simulink model "Integ_Model_Hepta"  (R2022a)
settings: configuration reference "VLS_Standard_Configuration" (kept outside this file)
undefined symbols (not defined in the file or in its folder): C_AFS_SpeedThrAct, C_AfsRampTimeMatrix, C_AnimationOnLoop, C_AnimationPeriod, C_AnimationPriority, C_CieCurveGammaToPwmY, C_CieCurvePwmToGammaY, C_CL_Ti_Speed_Hystresis, C_CL_Ti_Speed_Threshold, C_ClActAlgo, C_ClLeftSideTable_Alpha1, C_ClLeftSideTable_Alpha2, C_ClManeuverPwm, C_ClRightSideTable_Alpha1, C_ClRightSideTable_Alpha2, C_ClSpeedCurve, C_ClTableSize, C_ClTownPwm, C_Config, C_CSpeed0, C_DblDeadZone, C_DblEnable, C_DblInterDblAngValues, C_DblInterStwAngValues, C_DblLeftAngles, C_DblRampTime, C_DblRateLimit, C_DblRightAngles, C_DblSlavePeriod, C_DblSpeed0, C_DefaultValue, C_DrlRampTime, C_EndIndexOfEachLightingModule, C_EndValues, C_ForceExternalAfsMode, C_IndexOfStartStepForEachScenario, C_IsClOnTps, C_IsDblActive, C_IsDrlAutorizedInPower2, C_IsDrlPlOnTps, C_IsPlAutorizedInPower2, C_IsTiAutorizedInPower2, C_IsTiOnTps, C_LedCenterDist, C_LedCenterLimits, C_LedLeftDist, C_LedRightDist, C_LedStartIndexOfCl, C_LedStartIndexOfDrlPl, C_LedStartIndexOfTi, C_LeftDblMaxAngle, C_LeftDblMinAngle, C_MaintainAnimationPwm, C_MaintainAnimationTime, C_NumOfStepsForEachScenario, C_PlNominalPwm, C_PlOverDRL, C_RightDblMaxAngle, C_RightDblMinAngle, C_StartIndexOfEachLightingModule ... (+14)
libraries: simulink x11, AFS_MasterFeature x2, DodecaPreprocessingLib x1, Cl_Lib x1, DBL_MasterLib x1, AfsSlaveLib x1, DblSlaveLib x1, StdAnimationLibrary_R2020b x1, Ramp_Library_R2017b x1, STD_Signaling_Lib x1
(part 1 of 2)
settings Model: DataDictionary=Hepta_Integrated_SLDD.sldd  Creator=ahashem  LastModifiedBy=yli69
settings ConfigSetRef: SourceName=VLS_Standard_Configuration

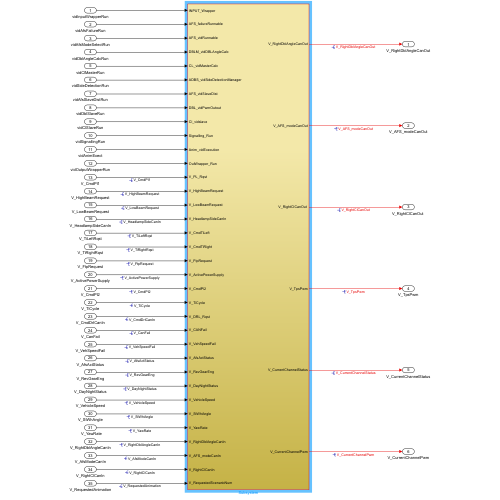
[thumbnail: Simulink's stored preview of the top-level diagram]
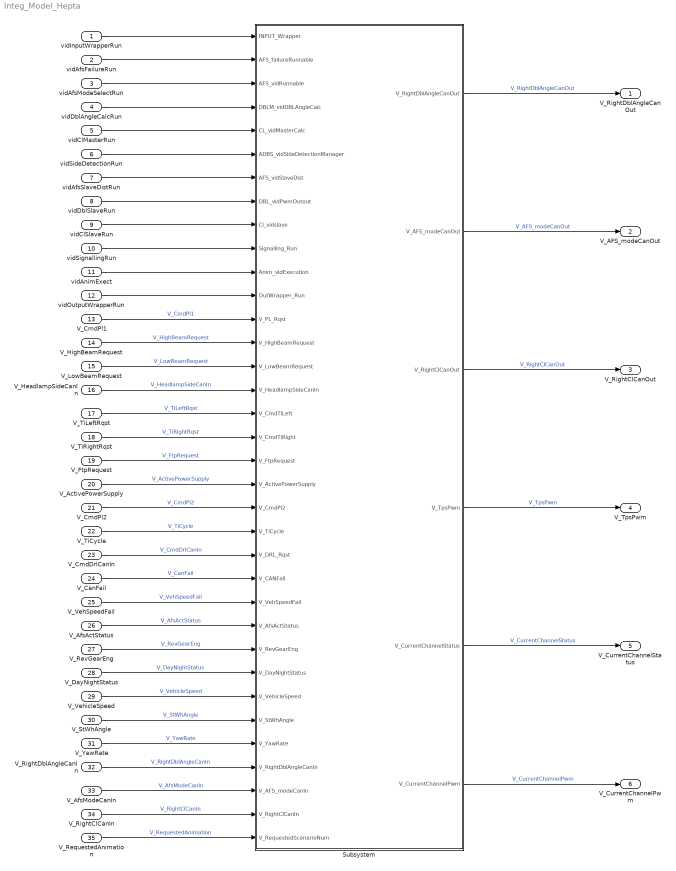
== system Integ_Model_Hepta ==
  vidInputWrapperRun : Inport  OutputFunctionCall=on
  vidAfsFailureRun : Inport  Port=2  OutputFunctionCall=on
  vidAfsModeSelectRun : Inport  Port=3  OutputFunctionCall=on
  vidDblAngleCalcRun : Inport  Port=4  SampleTime=0.02  OutputFunctionCall=on
  vidClMasterRun : Inport  Port=5  SampleTime=0.02  OutputFunctionCall=on
  vidSideDetectionRun : Inport  Port=6  OutputFunctionCall=on
  vidAfsSlaveDistRun : Inport  Port=7  OutputFunctionCall=on
  vidDblSlaveRun : Inport  Port=8  OutputFunctionCall=on
  vidClSlaveRun : Inport  Port=9  OutputFunctionCall=on
  vidSignallingRun : Inport  Port=10  OutputFunctionCall=on
  vidAnimExect : Inport  Port=11  OutputFunctionCall=on
  vidOutputWrapperRun : Inport  Port=12  OutputFunctionCall=on
  V_CmdPl1 : Inport  Port=13
  V_HighBeamRequest : Inport  Port=14
  V_LowBeamRequest : Inport  Port=15
  V_HeadlampSideCanIn : Inport  Port=16
  V_TiLeftRqst : Inport  Port=17
  V_TiRightRqst : Inport  Port=18
  V_FtpRequest : Inport  Port=19
  V_ActivePowerSupply : Inport  Port=20
  V_CmdPl2 : Inport  Port=21
  V_TiCycle : Inport  Port=22
  V_CmdDrlCanIn : Inport  Port=23
  V_CanFail : Inport  Port=24
  V_VehSpeedFail : Inport  Port=25
  V_AfsActStatus : Inport  Port=26
  V_RevGearEng : Inport  Port=27
  V_DayNightStatus : Inport  Port=28
  V_VehicleSpeed : Inport  Port=29
  V_StWhAngle : Inport  Port=30
  "  V_YawRate" : Inport  Port=31
  V_RightDblAngleCanIn : Inport  Port=32
  V_AfsModeCanIn : Inport  Port=33
  V_RightClCanIn : Inport  Port=34
  V_RequestedAnimation : Inport  Port=35
  Subsystem : Subsystem
  V_RightDblAngleCanOut : Outport  VectorParamsAs1DForOutWhenUnconnected=off
  V_AFS_modeCanOut : Outport  Port=2  VectorParamsAs1DForOutWhenUnconnected=off
  "V_RightClCanOut " : Outport  Port=3  VectorParamsAs1DForOutWhenUnconnected=off
  V_TpsPwm : Outport  Port=4
  V_CurrentChannelStatus : Outport  Port=5
  V_CurrentChannelPwm : Outport  Port=6
  wires:
  vidSignallingRun/1 -> Subsystem/10(Signalling_Run)
  vidInputWrapperRun/1 -> Subsystem/1(INPUT_Wrapper)
  vidAfsSlaveDistRun/1 -> Subsystem/7(AFS_vidSlaveDist)
  V_CmdPl1/1 -> Subsystem/13(V_PL_Rqst)  "V_CmdPl1"
  V_CmdDrlCanIn/1 -> Subsystem/23(V_DRL_Rqst)  "V_CmdDrlCanIn"
  V_HighBeamRequest/1 -> Subsystem/14(V_HighBeamRequest)  "V_HighBeamRequest"
  V_LowBeamRequest/1 -> Subsystem/15(V_LowBeamRequest)  "V_LowBeamRequest"
  vidDblSlaveRun/1 -> Subsystem/8(DBL_vidPwmOutout)
  V_HeadlampSideCanIn/1 -> Subsystem/16(V_HeadlampSideCanIn)  "V_HeadlampSideCanIn"
  V_TiRightRqst/1 -> Subsystem/18(V_CmdTiRight)  "V_TiRightRqst"
  V_TiLeftRqst/1 -> Subsystem/17(V_CmdTiLeft)  "V_TiLeftRqst"
  V_FtpRequest/1 -> Subsystem/19(V_FtpRequest)  "V_FtpRequest"
  V_ActivePowerSupply/1 -> Subsystem/20(V_ActivePowerSupply)  "V_ActivePowerSupply"
  V_TiCycle/1 -> Subsystem/22(V_TiCycle)  "V_TiCycle"
  V_CmdPl2/1 -> Subsystem/21(V_CmdPl2)  "V_CmdPl2"
  vidOutputWrapperRun/1 -> Subsystem/12(OutWrapper_Run)
  vidSideDetectionRun/1 -> Subsystem/6(ADBS_vidSideDetectionManager)
  vidAfsFailureRun/1 -> Subsystem/2(AFS_failureRunnable)
  vidAfsModeSelectRun/1 -> Subsystem/3(AFS_vidRunnable)
  vidDblAngleCalcRun/1 -> Subsystem/4(DBLM_vidDBLAngleCalc)
  V_CanFail/1 -> Subsystem/24(V_CANFail)  "V_CanFail"
  V_VehSpeedFail/1 -> Subsystem/25(V_VehSpeedFail)  "V_VehSpeedFail"
  V_AfsActStatus/1 -> Subsystem/26(V_AfsActStatus)  "V_AfsActStatus"
  V_RevGearEng/1 -> Subsystem/27(V_RevGearEng)  "V_RevGearEng"
  V_DayNightStatus/1 -> Subsystem/28(V_DayNightStatus)  "V_DayNightStatus"
  V_AfsModeCanIn/1 -> Subsystem/33(V_AFS_modeCanIn)  "V_AfsModeCanIn"
  V_RightDblAngleCanIn/1 -> Subsystem/32(V_RightDblAngleCanIn)  "V_RightDblAngleCanIn"
  V_VehicleSpeed/1 -> Subsystem/29(V_VehicleSpeed)  "V_VehicleSpeed"
  V_StWhAngle/1 -> Subsystem/30(V_StWhAngle)  "V_StWhAngle"
  "  V_YawRate"/1 -> Subsystem/31(V_YawRate)  "V_YawRate"
  Subsystem/2(V_AFS_modeCanOut) -> V_AFS_modeCanOut/1  "V_AFS_modeCanOut"
  Subsystem/1(V_RightDblAngleCanOut) -> V_RightDblAngleCanOut/1  "V_RightDblAngleCanOut"
  vidClMasterRun/1 -> Subsystem/5(CL_vidMasterCalc)
  vidClSlaveRun/1 -> Subsystem/9(Cl_vidslave)
  V_RightClCanIn/1 -> Subsystem/34(V_RightClCanIn)  "V_RightClCanIn"
  Subsystem/3("V_RightClCanOut ") -> "V_RightClCanOut "/1  "V_RightClCanOut"
  Subsystem/4(V_TpsPwm) -> V_TpsPwm/1  "V_TpsPwm"
  Subsystem/5(V_CurrentChannelStatus) -> V_CurrentChannelStatus/1  "V_CurrentChannelStatus"
  Subsystem/6(V_CurrentChannelPwm) -> V_CurrentChannelPwm/1  "V_CurrentChannelPwm"
  vidAnimExect/1 -> Subsystem/11(Anim_vidExecution)
  V_RequestedAnimation/1 -> Subsystem/35(V_RequestedScenarioNum)  "V_RequestedAnimation"

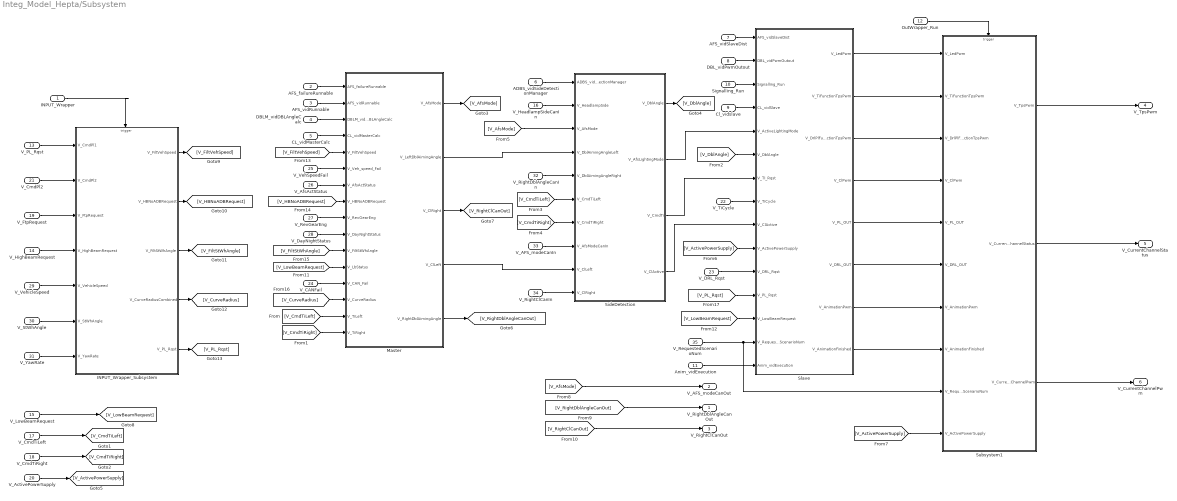
== system Integ_Model_Hepta/Subsystem ==
  INPUT_Wrapper : Inport
  AFS_failureRunnable : Inport  Port=2  OutputFunctionCall=on
  AFS_vidRunnable : Inport  Port=3  OutputFunctionCall=on
  DBLM_vidDBLAngleCalc : Inport  Port=4  SampleTime=0.02  OutputFunctionCall=on
  CL_vidMasterCalc : Inport  Port=5  SampleTime=0.02  OutputFunctionCall=on
  ADBS_vidSideDetectionManager : Inport  Port=6
  AFS_vidSlaveDist : Inport  Port=7
  DBL_vidPwmOutout : Inport  Port=8
  Cl_vidslave : Inport  Port=9
  Signalling_Run : Inport  Port=10
  Anim_vidExecution : Inport  Port=11
  OutWrapper_Run : Inport  Port=12
  V_PL_Rqst : Inport  Port=13
  V_HighBeamRequest : Inport  Port=14
  V_LowBeamRequest : Inport  Port=15
  V_HeadlampSideCanIn : Inport  Port=16
  V_CmdTiLeft : Inport  Port=17
  V_CmdTiRight : Inport  Port=18
  V_FtpRequest : Inport  Description=|  Port=19
      | Requirements:
      | Covers{PAKU_YRS_2769}
  V_ActivePowerSupply : Inport  Port=20
  V_CmdPl2 : Inport  Port=21
  V_TiCycle : Inport  Port=22
  V_DRL_Rqst : Inport  Port=23
  V_CANFail : Inport  Port=24
  V_VehSpeedFail : Inport  Port=25
  V_AfsActStatus : Inport  Port=26
  V_RevGearEng : Inport  Port=27
  V_DayNightStatus : Inport  Port=28
  V_VehicleSpeed : Inport  Port=29
  V_StWhAngle : Inport  Port=30
  V_YawRate : Inport  Port=31
  V_RightDblAngleCanIn : Inport  Port=32
  V_AFS_modeCanIn : Inport  Port=33
  V_RightClCanIn : Inport  Port=34
  V_RequestedScenarioNum : Inport  Port=35
  INPUT_Wrapper_Subsystem : Subsystem  Description=Clustering subsystem
  Master : Subsystem
  SideDetection : Subsystem
  Slave : Subsystem
  Subsystem1 : Subsystem
  V_RightDblAngleCanOut : Outport  VectorParamsAs1DForOutWhenUnconnected=off
  V_AFS_modeCanOut : Outport  Port=2  VectorParamsAs1DForOutWhenUnconnected=off
  "V_RightClCanOut " : Outport  Port=3  VectorParamsAs1DForOutWhenUnconnected=off
  V_TpsPwm : Outport  Port=4
  V_CurrentChannelStatus : Outport  Port=5
  V_CurrentChannelPwm : Outport  Port=6
  wires:
  V_LowBeamRequest/1 -> [V_LowBeamRequest]
  INPUT_Wrapper/1 -> INPUT_Wrapper_Subsystem/Trigger
  AFS_vidSlaveDist/1 -> Slave/1(AFS_vidSlaveDist)
  DBL_vidPwmOutout/1 -> Slave/2(DBL_vidPwmOutout)
  V_FtpRequest/1 -> INPUT_Wrapper_Subsystem/3(V_FtpRequest)
  V_HeadlampSideCanIn/1 -> SideDetection/2(V_HeadlampSide)
  V_CmdTiLeft/1 -> [V_CmdTiLeft]
  SideDetection/3(V_CmdTi) -> Slave/7(V_TI_Rqst)
  Slave/2(V_TiFunctionTpsPwm) -> Subsystem1/2(V_TiFunctionTpsPwm)
  Slave/3(V_DrlPlFunctionTpsPwm) -> Subsystem1/3(V_DrlPlFunctionTpsPwm)
  V_PL_Rqst/1 -> INPUT_Wrapper_Subsystem/1(V_CmdPl1)
  V_CmdPl2/1 -> INPUT_Wrapper_Subsystem/2(V_CmdPl2)
  OutWrapper_Run/1 -> Subsystem1/Trigger
  V_DRL_Rqst/1 -> Slave/11(V_DRL_Rqst)
  V_TiCycle/1 -> Slave/8(V_TiCycle)
  Signalling_Run/1 -> Slave/3(Signalling_Run)
  Slave/1(V_LedPwm) -> Subsystem1/1(V_LedPwm)
  ADBS_vidSideDetectionManager/1 -> SideDetection/1(ADBS_vidSideDetectionManager)
  Master/2(V_LeftDblAimingAngle) -> SideDetection/4(V_DblAimingAngleLeft)
  AFS_vidRunnable/1 -> Master/2(AFS_vidRunnable)
  AFS_failureRunnable/1 -> Master/1(AFS_failureRunnable)
  DBLM_vidDBLAngleCalc/1 -> Master/3(DBLM_vidDBLAngleCalc)
  V_AfsActStatus/1 -> Master/7(V_AfsActStatus)
  V_DayNightStatus/1 -> Master/10(V_DayNightStatus)
  V_CANFail/1 -> Master/13(V_CAN_Fail)
  V_VehSpeedFail/1 -> Master/6(V_Veh_speed_Fail)
  V_RevGearEng/1 -> Master/9(V_RevGearEng)
  V_HighBeamRequest/1 -> INPUT_Wrapper_Subsystem/4(V_HighBeamRequest)
  Master/1(V_AfsMode) -> [V_AfsMode]
  SideDetection/2(V_AfsLightingMode) -> Slave/5(V_ActiveLightingMode)
  V_RightDblAngleCanIn/1 -> SideDetection/5(V_DblAimingAngleRight)
  V_AFS_modeCanIn/1 -> SideDetection/8(V_AfsModeCanIn)
  V_StWhAngle/1 -> INPUT_Wrapper_Subsystem/6(V_StWhAngle)
  V_YawRate/1 -> INPUT_Wrapper_Subsystem/7(V_YawRate)
  V_VehicleSpeed/1 -> INPUT_Wrapper_Subsystem/5(V_VehicleSpeed)
  Master/4(V_ClLeft) -> SideDetection/9(V_ClLeft)
  V_RightClCanIn/1 -> SideDetection/10(V_ClRight)
  SideDetection/4(V_ClActive) -> Slave/9(V_ClActive)
  Cl_vidslave/1 -> Slave/4(CL_vidSlave)
  CL_vidMasterCalc/1 -> Master/4(CL_vidMasterCalc)
  V_CmdTiRight/1 -> [V_CmdTiRight]
  [V_CmdTiLeft] -> Master/15(V_TiLeft)
  [V_CmdTiRight] -> Master/16(V_TiRight)
  [V_AfsMode] -> SideDetection/3(V_AfsMode)
  [V_CmdTiLeft] -> SideDetection/6(V_CmdTiLeft)
  [V_CmdTiRight] -> SideDetection/7(V_CmdTiRight)
  SideDetection/1(V_DblAngle) -> [V_DblAngle]
  [V_DblAngle] -> Slave/6(V_DblAngle)
  V_ActivePowerSupply/1 -> [V_ActivePowerSupply]
  [V_ActivePowerSupply] -> Slave/10(V_ActivePowerSupply)
  [V_ActivePowerSupply] -> Subsystem1/10(V_ActivePowerSupply)
  [V_AfsMode] -> V_AFS_modeCanOut/1
  Master/5(V_RightDblAimingAngle) -> [V_RightDblAngleCanOut]
  [V_RightDblAngleCanOut] -> V_RightDblAngleCanOut/1
  Master/3(V_ClRight) -> [V_RightClCanOut]
  [V_RightClCanOut] -> "V_RightClCanOut "/1
  Subsystem1/3(V_CurrentChannelPwm) -> V_CurrentChannelPwm/1
  Subsystem1/2(V_CurrentChannelStatus) -> V_CurrentChannelStatus/1
  Subsystem1/1(V_TpsPwm) -> V_TpsPwm/1
  Slave/5(V_PL_OUT) -> Subsystem1/5(V_PL_OUT)
  Slave/6(V_DRL_OUT) -> Subsystem1/6(V_DRL_OUT)
  Slave/4(V_ClPwm) -> Subsystem1/4(V_ClPwm)
  [V_LowBeamRequest] -> Master/12(V_LbStatus)
  [V_LowBeamRequest] -> Slave/13(V_LowBeamRequest)
  Anim_vidExecution/1 -> Slave/15(Anim_vidExecution)
  Slave/7(V_AnimationPwm) -> Subsystem1/7(V_AnimationPwm)
  Slave/8(V_AnimationFinished) -> Subsystem1/8(V_AnimationFinished)
  V_RequestedScenarioNum/1 -> Subsystem1/9(V_RequestedScenarioNum), Slave/14(V_RequestedScenarioNum)
  INPUT_Wrapper_Subsystem/1(V_FiltVehSpeed) -> [V_FiltVehSpeed]
  [V_FiltVehSpeed] -> Master/5(V_FiltVehSpeed)
  INPUT_Wrapper_Subsystem/2(V_HBNoADBRequest) -> [V_HBNoADBRequest]
  [V_HBNoADBRequest] -> Master/8(V_HBNoADBRequest)
  INPUT_Wrapper_Subsystem/3(V_FiltStWhAngle) -> [V_FiltStWhAngle]
  [V_FiltStWhAngle] -> Master/11(V_FiltStWhAngle)
  INPUT_Wrapper_Subsystem/4(V_CurveRadiusCombined) -> [V_CurveRadius]
  [V_CurveRadius] -> Master/14(V_CurveRadius)
  INPUT_Wrapper_Subsystem/5(V_PL_Rqst) -> [V_PL_Rqst]
  [V_PL_Rqst] -> Slave/12(V_PL_Rqst)

== system Integ_Model_Hepta/Subsystem/INPUT_Wrapper_Subsystem ==
  V_CmdPl1 : Inport
  V_CmdPl2 : Inport  Port=2
  V_FtpRequest : Inport  Port=3
  V_HighBeamRequest : Inport  Port=4
  V_VehicleSpeed : Inport  Port=5
  V_StWhAngle : Inport  Port=6
  V_YawRate : Inport  Port=7
  function : TriggerPort  TriggerType=function-call  VariantControl=Variant
      settings: AttributesFormatString=StatesWhenEnabling: %<StatesWhenEnabling>
  DodecaPreprocessingLib : DodecaPreprocessingLib/DodecaPreprocessingLib  SystemSampleTime=-1  VariantActivationTime=update diagram  Latency=0  AutoFrameSizeCalculation=off
  Logical Operator1 : Logic  Operator=OR  AllPortsSameDT=off  OutDataTypeStr=boolean
  Logical Operator2 : Logic  Operator=OR  AllPortsSameDT=off  OutDataTypeStr=boolean
  Terminator : Terminator
  Terminator1 : Terminator
  Terminator2 : Terminator
  V_FiltVehSpeed : Outport  VectorParamsAs1DForOutWhenUnconnected=off
  V_HBNoADBRequest : Outport  Port=2
  V_FiltStWhAngle : Outport  Port=3  VectorParamsAs1DForOutWhenUnconnected=off
  V_CurveRadiusCombined : Outport  Port=4  VectorParamsAs1DForOutWhenUnconnected=off
  V_PL_Rqst : Outport  Port=5
  wires:
  V_CmdPl1/1 -> Logical Operator2/1
  V_CmdPl2/1 -> Logical Operator2/2
  Logical Operator2/1 -> V_PL_Rqst/1
  V_FtpRequest/1 -> Logical Operator1/1
  V_HighBeamRequest/1 -> Logical Operator1/2
  Logical Operator1/1 -> V_HBNoADBRequest/1
  V_VehicleSpeed/1 -> DodecaPreprocessingLib/1
  V_StWhAngle/1 -> DodecaPreprocessingLib/2
  V_YawRate/1 -> DodecaPreprocessingLib/3
  DodecaPreprocessingLib/3 -> Terminator/1
  DodecaPreprocessingLib/4 -> Terminator1/1
  DodecaPreprocessingLib/5 -> Terminator2/1
  DodecaPreprocessingLib/2 -> V_FiltStWhAngle/1
  DodecaPreprocessingLib/1 -> V_FiltVehSpeed/1
  DodecaPreprocessingLib/6 -> V_CurveRadiusCombined/1

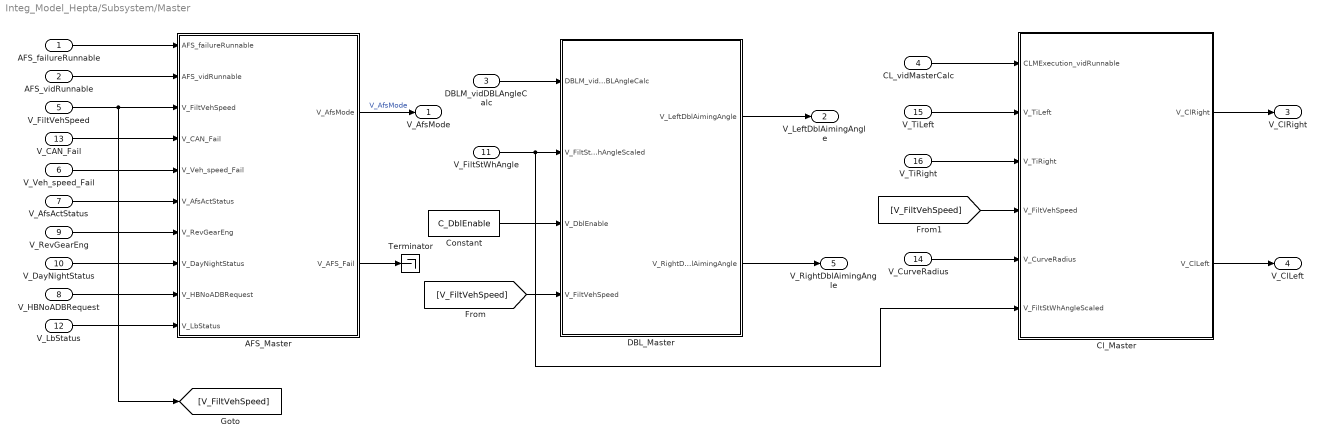
== system Integ_Model_Hepta/Subsystem/Master ==
  AFS_failureRunnable : Inport  OutputFunctionCall=on
  AFS_vidRunnable : Inport  Port=2  OutputFunctionCall=on
  DBLM_vidDBLAngleCalc : Inport  Port=3  SampleTime=0.02  OutputFunctionCall=on
  CL_vidMasterCalc : Inport  Port=4  SampleTime=0.02  OutputFunctionCall=on
  V_FiltVehSpeed : Inport  Port=5
  V_Veh_speed_Fail : Inport  Port=6
  V_AfsActStatus : Inport  Port=7
  V_HBNoADBRequest : Inport  Port=8
  V_RevGearEng : Inport  Port=9
  V_DayNightStatus : Inport  Port=10
  V_FiltStWhAngle : Inport  Port=11
  V_LbStatus : Inport  Port=12
  V_CAN_Fail : Inport  Port=13
  V_CurveRadius : Inport  Port=14
  V_TiLeft : Inport  Port=15
  V_TiRight : Inport  Port=16
  AFS_Master : Subsystem
  Cl_Master : Subsystem
  Constant : Constant  Value=C_DblEnable  OutDataTypeStr=Inherit: Inherit via back propagation
  DBL_Master : Subsystem
  Terminator : Terminator
  V_AfsMode : Outport  PortDimensions=1
  V_LeftDblAimingAngle : Outport  Port=2  VectorParamsAs1DForOutWhenUnconnected=off
  V_ClRight : Outport  Port=3
  V_ClLeft : Outport  Port=4
  V_RightDblAimingAngle : Outport  Port=5  VectorParamsAs1DForOutWhenUnconnected=off
  wires:
  AFS_Master/2(V_AFS_Fail) -> Terminator/1
  AFS_Master/1(V_AfsMode) -> V_AfsMode/1  "V_AfsMode"
  AFS_failureRunnable/1 -> AFS_Master/1(AFS_failureRunnable)
  AFS_vidRunnable/1 -> AFS_Master/2(AFS_vidRunnable)
  V_FiltVehSpeed/1 -> [V_FiltVehSpeed], AFS_Master/3(V_FiltVehSpeed)
  V_CAN_Fail/1 -> AFS_Master/4(V_CAN_Fail)
  V_Veh_speed_Fail/1 -> AFS_Master/5(V_Veh_speed_Fail)
  V_AfsActStatus/1 -> AFS_Master/6(V_AfsActStatus)
  V_FiltStWhAngle/1 -> Cl_Master/6(V_FiltStWhAngleScaled), DBL_Master/2(V_FiltStWhAngleScaled)
  Constant/1 -> DBL_Master/3(V_DblEnable)
  DBLM_vidDBLAngleCalc/1 -> DBL_Master/1(DBLM_vidDBLAngleCalc)
  DBL_Master/1(V_LeftDblAimingAngle) -> V_LeftDblAimingAngle/1
  DBL_Master/2(V_RightDblAimingAngle) -> V_RightDblAimingAngle/1
  Cl_Master/2(V_ClLeft) -> V_ClLeft/1
  V_TiLeft/1 -> Cl_Master/2(V_TiLeft)
  CL_vidMasterCalc/1 -> Cl_Master/1(CLMExecution_vidRunnable)
  V_TiRight/1 -> Cl_Master/3(V_TiRight)
  V_CurveRadius/1 -> Cl_Master/5(V_CurveRadius)
  Cl_Master/1(V_ClRight) -> V_ClRight/1
  V_RevGearEng/1 -> AFS_Master/7(V_RevGearEng)
  V_DayNightStatus/1 -> AFS_Master/8(V_DayNightStatus)
  V_HBNoADBRequest/1 -> AFS_Master/9(V_HBNoADBRequest)
  V_LbStatus/1 -> AFS_Master/10(V_LbStatus)
  [V_FiltVehSpeed] -> DBL_Master/4(V_FiltVehSpeed)
  [V_FiltVehSpeed] -> Cl_Master/4(V_FiltVehSpeed)

== system Integ_Model_Hepta/Subsystem/SideDetection ==
  ADBS_vidSideDetectionManager : Inport
  V_HeadlampSide : Inport  Port=2
  V_AfsMode : Inport  Port=3
  V_DblAimingAngleLeft : Inport  Port=4
  V_DblAimingAngleRight : Inport  Port=5
  V_CmdTiLeft : Inport  Port=6
  V_CmdTiRight : Inport  Port=7
  V_AfsModeCanIn : Inport  Port=8
  V_ClLeft : Inport  Port=9
  V_ClRight : Inport  Port=10
  SideDetectionManager : Subsystem  Description=|
      | Requirements:
      | Covers{PAKU_YRS_2708,PAKU_YRS_2758,PAKU_YRS_2734,PAKU_YRS_2753,PAKU_YRS_2783}
  V_DblAngle : Outport
  V_AfsLightingMode : Outport  Port=2
  V_CmdTi : Outport  Port=3
  V_ClActive : Outport  Port=4
  wires:
  ADBS_vidSideDetectionManager/1 -> SideDetectionManager/Trigger
  V_HeadlampSide/1 -> SideDetectionManager/1(V_HeadlampSide)
  V_DblAimingAngleLeft/1 -> SideDetectionManager/2(V_DblAimingAngleLeft)
  V_CmdTiLeft/1 -> SideDetectionManager/4(V_CmdTiLeft)
  V_DblAimingAngleRight/1 -> SideDetectionManager/3(V_DblAimingAngleRight)
  V_CmdTiRight/1 -> SideDetectionManager/5(V_CmdTiRight)
  SideDetectionManager/2(V_DblAngle) -> V_DblAngle/1
  SideDetectionManager/3(V_CmdTi) -> V_CmdTi/1
  V_AfsMode/1 -> SideDetectionManager/6(V_AfsMode)
  V_AfsModeCanIn/1 -> SideDetectionManager/7(V_AfsModeCanIn)
  SideDetectionManager/1(V_AfsLightingMode) -> V_AfsLightingMode/1
  V_ClLeft/1 -> SideDetectionManager/8(V_ClLeft)
  V_ClRight/1 -> SideDetectionManager/9(V_ClRight)
  SideDetectionManager/4(V_ClActive) -> V_ClActive/1

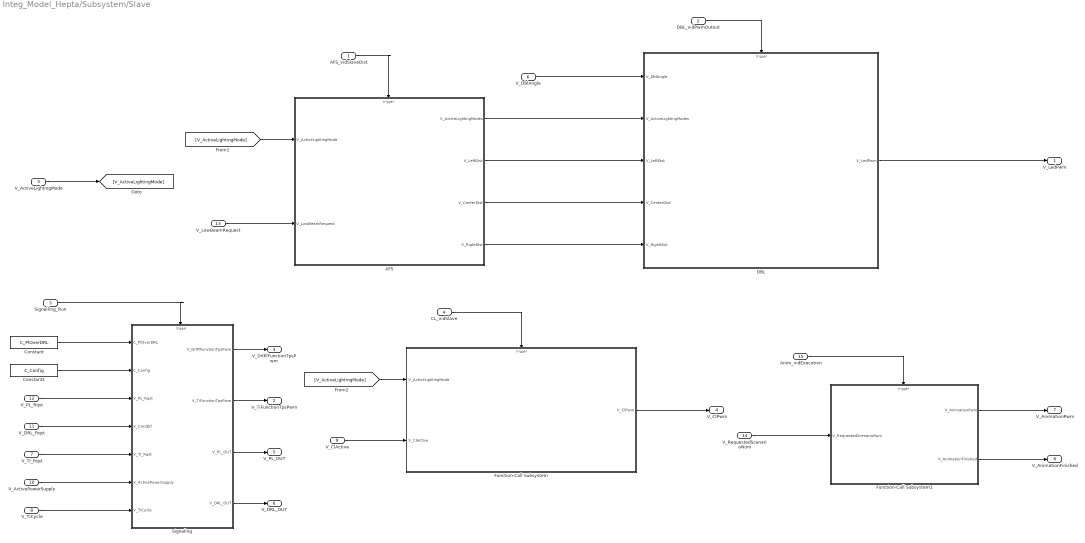
== system Integ_Model_Hepta/Subsystem/Slave ==
  AFS_vidSlaveDist : Inport
  DBL_vidPwmOutout : Inport  Port=2
  Signalling_Run : Inport  Port=3
  CL_vidSlave : Inport  Port=4
  V_ActiveLightingMode : Inport  Port=5
  V_DblAngle : Inport  Port=6
  V_TI_Rqst : Inport  Port=7
  V_TiCycle : Inport  Port=8
  V_ClActive : Inport  Port=9
  V_ActivePowerSupply : Inport  Port=10
  V_DRL_Rqst : Inport  Port=11
  V_PL_Rqst : Inport  Port=12
  V_LowBeamRequest : Inport  Port=13
  V_RequestedScenarioNum : Inport  Port=14
  Anim_vidExecution : Inport  Port=15
  AFS : Subsystem
  Constant : Constant  Value=C_PlOverDRL
  Constant1 : Constant  Value=C_Config
  DBL : Subsystem  Description=Clustering subsystem
  Function-Call Subsystem : Subsystem  TreatAsAtomicUnit=on
  Function-Call Subsystem1 : Subsystem  TreatAsAtomicUnit=on
  Signaling : Subsystem  Description=/* 2ST220085-0210-635_CYRS_P2_Hepta_Platform: S____2287 V02 */
  V_LedPwm : Outport  VectorParamsAs1DForOutWhenUnconnected=off
  V_TiFunctionTpsPwm : Outport  Port=2
  V_DrlPlFunctionTpsPwm : Outport  Port=3
  V_ClPwm : Outport  Port=4
  V_PL_OUT : Outport  Port=5
  V_DRL_OUT : Outport  Port=6
  V_AnimationPwm : Outport  Port=7  VectorParamsAs1DForOutWhenUnconnected=off
  V_AnimationFinished : Outport  Port=8  VectorParamsAs1DForOutWhenUnconnected=off
  wires:
  V_TiCycle/1 -> Signaling/7(V_TiCycle)
  Constant/1 -> Signaling/1(C_PlOverDRL)
  Constant1/1 -> Signaling/2(C_Config)
  V_ActivePowerSupply/1 -> Signaling/6(V_ActivePowerSupply)
  Signalling_Run/1 -> Signaling/Trigger
  V_TI_Rqst/1 -> Signaling/5(V_TI_Rqst)
  V_PL_Rqst/1 -> Signaling/3(V_PL_Rqst)
  V_DRL_Rqst/1 -> Signaling/4(V_CmdDrl)
  Signaling/1(V_DrlPlFunctionTpsPwm) -> V_DrlPlFunctionTpsPwm/1
  Signaling/2(V_TiFunctionTpsPwm) -> V_TiFunctionTpsPwm/1
  V_DblAngle/1 -> DBL/1(V_DblAngle)
  AFS/2(V_LeftDist) -> DBL/3(V_LeftDist)
  [V_ActiveLightingMode] -> AFS/1(V_ActiveLightingMode)
  AFS/4(V_RightDist) -> DBL/5(V_RightDist)
  AFS_vidSlaveDist/1 -> AFS/Trigger
  AFS/3(V_CenterDist) -> DBL/4(V_CenterDist)
  AFS/1(V_ActiveLightingModes) -> DBL/2(V_ActiveLightingModes)
  DBL/1(V_LedPwm) -> V_LedPwm/1
  DBL_vidPwmOutout/1 -> DBL/Trigger
  V_ActiveLightingMode/1 -> [V_ActiveLightingMode]
  V_ClActive/1 -> Function-Call Subsystem/2(V_ClActive)
  [V_ActiveLightingMode] -> Function-Call Subsystem/1(V_ActiveLightingMode)
  CL_vidSlave/1 -> Function-Call Subsystem/Trigger
  Function-Call Subsystem/1(V_ClPwm) -> V_ClPwm/1
  Signaling/4(V_DRL_OUT) -> V_DRL_OUT/1
  Signaling/3(V_PL_OUT) -> V_PL_OUT/1
  V_LowBeamRequest/1 -> AFS/2(V_LowBeamRequest)
  V_RequestedScenarioNum/1 -> Function-Call Subsystem1/1(V_RequestedScenarioNum)
  Anim_vidExecution/1 -> Function-Call Subsystem1/Trigger
  Function-Call Subsystem1/1(V_AnimationPwm) -> V_AnimationPwm/1
  Function-Call Subsystem1/2(V_AnimationFinished) -> V_AnimationFinished/1

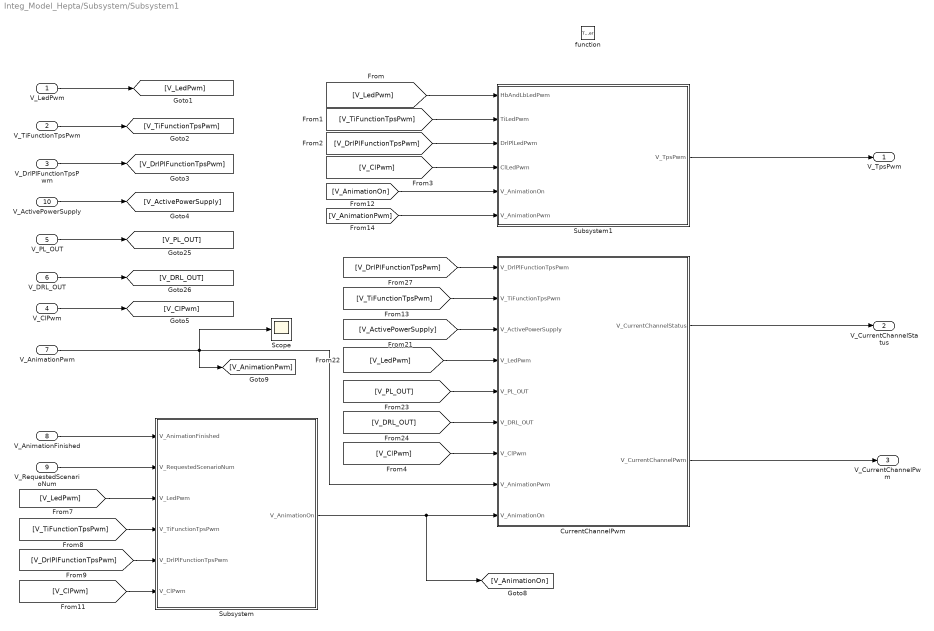
== system Integ_Model_Hepta/Subsystem/Subsystem1 ==
  V_LedPwm : Inport
  V_TiFunctionTpsPwm : Inport  Port=2
  V_DrlPlFunctionTpsPwm : Inport  Port=3
  V_ClPwm : Inport  Port=4
  V_PL_OUT : Inport  Port=5
  V_DRL_OUT : Inport  Port=6
  V_AnimationPwm : Inport  Port=7
  V_AnimationFinished : Inport  Port=8
  V_RequestedScenarioNum : Inport  Port=9
  V_ActivePowerSupply : Inport  Port=10
  function : TriggerPort  TriggerType=function-call  VariantControl=Variant
  CurrentChannelPwm : Subsystem
  Scope : Scope
  Subsystem : Subsystem
  Subsystem1 : Subsystem
  V_TpsPwm : Outport
  V_CurrentChannelStatus : Outport  Port=2
  V_CurrentChannelPwm : Outport  Port=3
  wires:
  [V_TiFunctionTpsPwm] -> CurrentChannelPwm/2(V_TiFunctionTpsPwm)
  V_PL_OUT/1 -> [V_PL_OUT]
  [V_PL_OUT] -> CurrentChannelPwm/5(V_PL_OUT)
  [V_DRL_OUT] -> CurrentChannelPwm/6(V_DRL_OUT)
  V_ActivePowerSupply/1 -> [V_ActivePowerSupply]
  V_DrlPlFunctionTpsPwm/1 -> [V_DrlPlFunctionTpsPwm]
  [V_LedPwm] -> CurrentChannelPwm/4(V_LedPwm)
  V_TiFunctionTpsPwm/1 -> [V_TiFunctionTpsPwm]
  V_DRL_OUT/1 -> [V_DRL_OUT]
  [V_ActivePowerSupply] -> CurrentChannelPwm/3(V_ActivePowerSupply)
  V_LedPwm/1 -> [V_LedPwm]
  [V_DrlPlFunctionTpsPwm] -> CurrentChannelPwm/1(V_DrlPlFunctionTpsPwm)
  V_ClPwm/1 -> [V_ClPwm]
  [V_ClPwm] -> CurrentChannelPwm/7(V_ClPwm)
  [V_ClPwm] -> Subsystem/6(V_ClPwm)
  [V_TiFunctionTpsPwm] -> Subsystem/4(V_TiFunctionTpsPwm)
  [V_LedPwm] -> Subsystem/3(V_LedPwm)
  [V_DrlPlFunctionTpsPwm] -> Subsystem/5(V_DrlPlFunctionTpsPwm)
  V_AnimationFinished/1 -> Subsystem/1(V_AnimationFinished)
  V_RequestedScenarioNum/1 -> Subsystem/2(V_RequestedScenarioNum)
  Subsystem/1(V_AnimationOn) -> [V_AnimationOn], CurrentChannelPwm/9(V_AnimationOn)
  V_AnimationPwm/1 -> Scope/1, [V_AnimationPwm], CurrentChannelPwm/8(V_AnimationPwm)
  [V_LedPwm] -> Subsystem1/1(HbAndLbLedPwm)
  [V_TiFunctionTpsPwm] -> Subsystem1/2(TiLedPwm)
  [V_DrlPlFunctionTpsPwm] -> Subsystem1/3(DrlPlLedPwm)
  [V_ClPwm] -> Subsystem1/4(ClLedPwm)
  [V_AnimationOn] -> Subsystem1/5(V_AnimationOn)
  [V_AnimationPwm] -> Subsystem1/6(V_AnimationPwm)
  Subsystem1/1(V_TpsPwm) -> V_TpsPwm/1
  CurrentChannelPwm/2(V_CurrentChannelPwm) -> V_CurrentChannelPwm/1
  CurrentChannelPwm/1(V_CurrentChannelStatus) -> V_CurrentChannelStatus/1

== system Integ_Model_Hepta/Subsystem/Master/AFS_Master ==
  AFS_failureRunnable : Inport  OutputFunctionCall=on
  AFS_vidRunnable : Inport  Port=2  OutputFunctionCall=on
  V_FiltVehSpeed : Inport  Port=3
  V_CAN_Fail : Inport  Port=4
  V_Veh_speed_Fail : Inport  Port=5
  V_AfsActStatus : Inport  Port=6
  V_RevGearEng : Inport  Port=7
  V_DayNightStatus : Inport  Port=8
  V_HBNoADBRequest : Inport  Port=9
  V_LbStatus : Inport  Port=10
  AFS_Master : Subsystem  Description=AFS_Master
  Constant{,1..5} (6 alike) : Constant  Value=0  OutDataTypeStr=Inherit: Inherit via back propagation
  Constant6 : Constant  Value=C_ForceExternalAfsMode  OutDataTypeStr=Inherit: Inherit via back propagation
  Display : Display
  V_AfsMode : Outport  PortDimensions=1
  V_AFS_Fail : Outport  Port=2  VectorParamsAs1DForOutWhenUnconnected=off
  wires:
  AFS_failureRunnable/1 -> AFS_Master/1(AFS_failureRunnable)
  AFS_vidRunnable/1 -> AFS_Master/2(AFS_vidRunnable)
  V_AfsActStatus/1 -> AFS_Master/8(V_AFS_ActStatus)
  V_Veh_speed_Fail/1 -> AFS_Master/5(V_Veh_speed_Fail)
  V_FiltVehSpeed/1 -> AFS_Master/3(V_FiltVehSpeed)
  V_CAN_Fail/1 -> AFS_Master/4(V_CAN_Fail)
  Constant/1 -> AFS_Master/7(V_Mod_RightFail), AFS_Master/6(V_Mod_LeftFail)
  Constant1/1 -> AFS_Master/10(V_ExternalAfsMode)
  Constant2/1 -> AFS_Master/12(V_ActivateADBFeatures)
  Constant3/1 -> AFS_Master/13(V_WetDetection)
  Constant4/1 -> AFS_Master/14(V_TouristModeActivated)
  Constant5/1 -> AFS_Master/15(V_Foggy)
  V_DayNightStatus/1 -> AFS_Master/17(V_DayNightStatus)
  V_RevGearEng/1 -> AFS_Master/16(V_RevGearEng)
  V_HBNoADBRequest/1 -> AFS_Master/18(V_HBNoADBRequest)
  V_LbStatus/1 -> AFS_Master/11(V_LbStatus)
  AFS_Master/2(V_AFS_Fail) -> V_AFS_Fail/1
  AFS_Master/1(V_AfsMode) -> Display/1, V_AfsMode/1
  Constant6/1 -> AFS_Master/9(V_ForceExternalAfsMode)

== system Integ_Model_Hepta/Subsystem/Master/Cl_Master ==
  CLMExecution_vidRunnable : Inport  SampleTime=0.02  OutputFunctionCall=on
  V_TiLeft : Inport  Port=2
  V_TiRight : Inport  Port=3
  V_FiltVehSpeed : Inport  Port=4
  V_CurveRadius : Inport  Port=5
  V_FiltStWhAngleScaled : Inport  Port=6
  CL_MasterFunction : Subsystem
  V_ClRight : Outport
  V_ClLeft : Outport  Port=2
  wires:
  V_CurveRadius/1 -> CL_MasterFunction/4(V_CurveRadius)
  CLMExecution_vidRunnable/1 -> CL_MasterFunction/Trigger
  CL_MasterFunction/1(V_ClRight) -> V_ClRight/1
  V_FiltVehSpeed/1 -> CL_MasterFunction/3(V_FiltVehSpeed)
  CL_MasterFunction/2(V_ClLeft) -> V_ClLeft/1
  V_TiLeft/1 -> CL_MasterFunction/1(V_TiLeft)
  V_FiltStWhAngleScaled/1 -> CL_MasterFunction/5(V_FiltStWhAngleScaled)
  V_TiRight/1 -> CL_MasterFunction/2(V_TiRight)

== system Integ_Model_Hepta/Subsystem/Master/DBL_Master ==
  DBLM_vidDBLAngleCalc : Inport  SampleTime=0.02  OutputFunctionCall=on
  V_FiltStWhAngleScaled : Inport  Port=2
  V_DblEnable : Inport  Port=3
  V_FiltVehSpeed : Inport  Port=4
  Function-Call Subsystem : Subsystem  TreatAsAtomicUnit=on
  V_LeftDblAimingAngle : Outport  VectorParamsAs1DForOutWhenUnconnected=off
  V_RightDblAimingAngle : Outport  Port=2  VectorParamsAs1DForOutWhenUnconnected=off
  wires:
  DBLM_vidDBLAngleCalc/1 -> Function-Call Subsystem/Trigger
  V_DblEnable/1 -> Function-Call Subsystem/2(V_DblEnable)
  V_FiltStWhAngleScaled/1 -> Function-Call Subsystem/1(V_FiltStWhAngleScaled)
  V_FiltVehSpeed/1 -> Function-Call Subsystem/3(V_FiltVehSpeed)
  Function-Call Subsystem/1(V_LeftDblAimingAngle) -> V_LeftDblAimingAngle/1
  Function-Call Subsystem/2(V_RightDblAimingAngle) -> V_RightDblAimingAngle/1

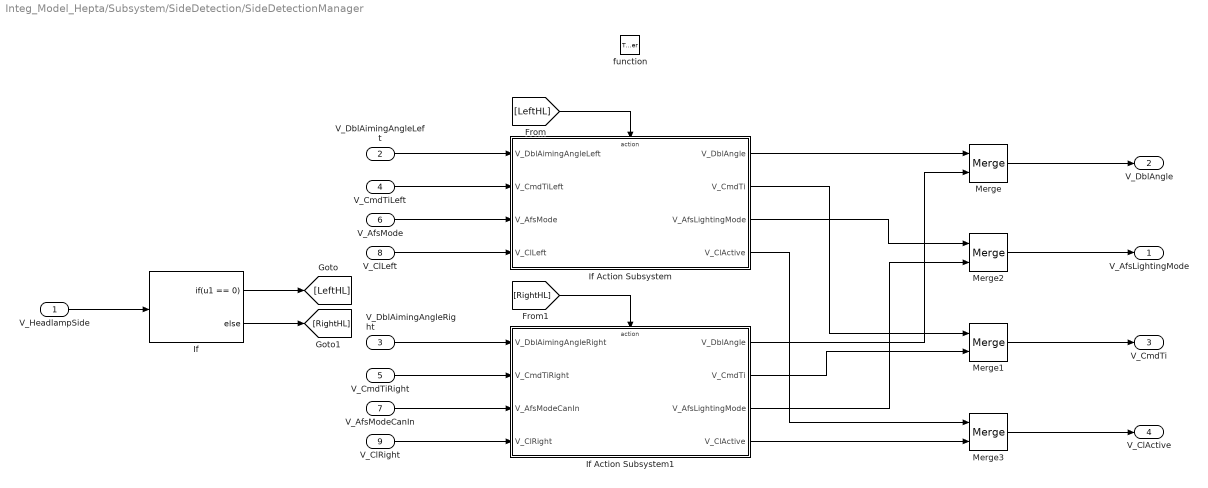
== system Integ_Model_Hepta/Subsystem/SideDetection/SideDetectionManager ==
  V_HeadlampSide : Inport
  V_DblAimingAngleLeft : Inport  Port=2
  V_DblAimingAngleRight : Inport  Port=3
  V_CmdTiLeft : Inport  Port=4
  V_CmdTiRight : Inport  Port=5
  V_AfsMode : Inport  Port=6
  V_AfsModeCanIn : Inport  Port=7
  V_ClLeft : Inport  Port=8
  V_ClRight : Inport  Port=9
  function : TriggerPort  TriggerType=function-call  VariantControl=Variant
  If : If  IfExpression=u1 == 0
  If Action Subsystem : Subsystem  TreatAsAtomicUnit=on
  If Action Subsystem1 : Subsystem  TreatAsAtomicUnit=on
  Merge{,1..3} (4 alike) : Merge
  V_AfsLightingMode : Outport
  V_DblAngle : Outport  Port=2
  V_CmdTi : Outport  Port=3
  V_ClActive : Outport  Port=4
  wires:
  V_HeadlampSide/1 -> If/1
  V_DblAimingAngleLeft/1 -> If Action Subsystem/1(V_DblAimingAngleLeft)
  V_CmdTiLeft/1 -> If Action Subsystem/2(V_CmdTiLeft)
  V_DblAimingAngleRight/1 -> If Action Subsystem1/1(V_DblAimingAngleRight)
  V_CmdTiRight/1 -> If Action Subsystem1/2(V_CmdTiRight)
  If Action Subsystem/1(V_DblAngle) -> Merge/1
  If Action Subsystem1/1(V_DblAngle) -> Merge/2
  If Action Subsystem/2(V_CmdTi) -> Merge1/1
  If Action Subsystem1/2(V_CmdTi) -> Merge1/2
  Merge/1 -> V_DblAngle/1
  If/1 -> [LeftHL]
  If/2 -> [RightHL]
  [LeftHL] -> If Action Subsystem/Action
  [RightHL] -> If Action Subsystem1/Action
  Merge1/1 -> V_CmdTi/1
  V_AfsMode/1 -> If Action Subsystem/3(V_AfsMode)
  V_AfsModeCanIn/1 -> If Action Subsystem1/3(V_AfsModeCanIn)
  If Action Subsystem/3(V_AfsLightingMode) -> Merge2/1
  If Action Subsystem1/3(V_AfsLightingMode) -> Merge2/2
  Merge2/1 -> V_AfsLightingMode/1
  V_ClLeft/1 -> If Action Subsystem/4(V_ClLeft)
  V_ClRight/1 -> If Action Subsystem1/4(V_ClRight)
  Merge3/1 -> V_ClActive/1
  If Action Subsystem/4(V_ClActive) -> Merge3/1
  If Action Subsystem1/4(V_ClActive) -> Merge3/2

== system Integ_Model_Hepta/Subsystem/Slave/AFS ==
  V_ActiveLightingMode : Inport
  V_LowBeamRequest : Inport  Port=2
  function : TriggerPort  TriggerType=function-call  VariantControl=Variant
      settings: AttributesFormatString=StatesWhenEnabling: %<StatesWhenEnabling>
  Constant : Constant  Value=C_LedLeftDist
  Constant1 : Constant  Value=C_LedCenterDist
  Constant2 : Constant  Value=C_LedRightDist
  Constant3 : Constant  Value=C_StartIndexOfEachLightingModule
  Constant4 : Constant  Value=C_CieCurvePwmToGammaY
  Constant5 : Constant  Value=C_CieCurveGammaToPwmY
  Constant6 : Constant  Value=C_DblSlavePeriod
  Constant7 : Constant  Value=C_EndIndexOfEachLightingModule
  Constant8 : Constant  Value=C_AfsRampTimeMatrix
  ConvertAfsModetoSlave : Subsystem
  LdAfsSlaveLib1 : AfsSlaveLib/LdAfsSlaveLib  SystemSampleTime=-1  VariantActivationTime=update diagram  Latency=0  AutoFrameSizeCalculation=off
  V_ActiveLightingModes : Outport
  V_LeftDist : Outport  Port=2
  V_CenterDist : Outport  Port=3
  V_RightDist : Outport  Port=4
  wires:
  Constant7/1 -> LdAfsSlaveLib1/6
  Constant/1 -> LdAfsSlaveLib1/2
  Constant6/1 -> LdAfsSlaveLib1/7
  Constant5/1 -> LdAfsSlaveLib1/9
  Constant8/1 -> LdAfsSlaveLib1/10
  Constant2/1 -> LdAfsSlaveLib1/4
  Constant3/1 -> LdAfsSlaveLib1/5
  Constant4/1 -> LdAfsSlaveLib1/8
  Constant1/1 -> LdAfsSlaveLib1/3
  LdAfsSlaveLib1/2 -> V_CenterDist/1
  LdAfsSlaveLib1/3 -> V_RightDist/1
  LdAfsSlaveLib1/1 -> V_LeftDist/1
  V_ActiveLightingMode/1 -> ConvertAfsModetoSlave/1(V_ActiveLightingMode)
  ConvertAfsModetoSlave/1(V_ActiveLightingModes) -> [V_ActiveLightingModes], LdAfsSlaveLib1/1
  [V_ActiveLightingModes] -> V_ActiveLightingModes/1
  V_LowBeamRequest/1 -> ConvertAfsModetoSlave/2(V_LowBeamRequest)

== system Integ_Model_Hepta/Subsystem/Slave/DBL ==
  V_DblAngle : Inport
  V_ActiveLightingModes : Inport  Port=2
  V_LeftDist : Inport  Port=3
  V_CenterDist : Inport  Port=4
  V_RightDist : Inport  Port=5
  function : TriggerPort  TriggerType=function-call  VariantControl=Variant
      settings: AttributesFormatString=StatesWhenEnabling: %<StatesWhenEnabling>
  Constant10 : Constant  Value=C_IsDblActive
  Constant11 : Constant  Value=C_DblLeftAngles
  Constant12 : Constant  Value=C_DblRightAngles
  Constant13 : Constant  Value=C_DblRampTime
  Constant14 : Constant  Value=C_LedCenterLimits
  Constant3 : Constant  Value=C_StartIndexOfEachLightingModule
  Constant4 : Constant  Value=C_CieCurvePwmToGammaY
  Constant5 : Constant  Value=C_CieCurveGammaToPwmY
  Constant6 : Constant  Value=C_DblSlavePeriod
  Constant7 : Constant  Value=C_EndIndexOfEachLightingModule
  LdDblSlaveLib : DblSlaveLib/LdDblSlaveLib  SystemSampleTime=-1  VariantActivationTime=update diagram  Latency=0  AutoFrameSizeCalculation=off
      link override DblCalc/ActiveModule/DblActive/MultiLed/Selector: IndexMode=One-based
  V_LedPwm : Outport  VectorParamsAs1DForOutWhenUnconnected=off
  wires:
  V_ActiveLightingModes/1 -> LdDblSlaveLib/1
  V_DblAngle/1 -> LdDblSlaveLib/2
  V_CenterDist/1 -> LdDblSlaveLib/4
  V_RightDist/1 -> LdDblSlaveLib/5
  V_LeftDist/1 -> LdDblSlaveLib/3
  LdDblSlaveLib/1 -> V_LedPwm/1
  Constant6/1 -> LdDblSlaveLib/13
  Constant4/1 -> LdDblSlaveLib/14
  Constant13/1 -> LdDblSlaveLib/12
  Constant5/1 -> LdDblSlaveLib/15
  Constant12/1 -> LdDblSlaveLib/11
  Constant11/1 -> LdDblSlaveLib/10
  Constant10/1 -> LdDblSlaveLib/9
  Constant7/1 -> LdDblSlaveLib/8
  Constant3/1 -> LdDblSlaveLib/7
  Constant14/1 -> LdDblSlaveLib/6

== system Integ_Model_Hepta/Subsystem/Slave/Function-Call Subsystem ==
  V_ActiveLightingMode : Inport
  V_ClActive : Inport  Port=2
  function : TriggerPort  TriggerType=function-call  VariantControl=Variant
  Constant1 : Constant  Value=C_ClTownPwm
  Constant2 : Constant  Value=N_E_Town
  Constant3 : Constant  Value=N_ManeuverMode
  Constant4 : Constant  Value=C_ClManeuverPwm
  Constant5 : Constant  Value=N_ClMaxPwm
  Constant6 : Constant  Value=N_Pwm_Off
  Equal : RelationalOperator  Operator===  OutDataTypeStr=boolean  RndMeth=Simplest  InputSameDT=off
  Equal1 : RelationalOperator  Operator===  OutDataTypeStr=boolean  RndMeth=Simplest  InputSameDT=off
  Switch : Switch  Criteria=u2 ~= 0  SaturateOnIntegerOverflow=off  InputSameDT=off
  Switch1 : Switch  Criteria=u2 ~= 0  SaturateOnIntegerOverflow=off  InputSameDT=off
  Switch2 : Switch  Criteria=u2 ~= 0  SaturateOnIntegerOverflow=off  InputSameDT=off
  V_ClPwm : Outport
  wires:
  V_ClActive/1 -> Switch/2
  Constant5/1 -> Switch/1
  Switch/1 -> V_ClPwm/1
  Switch1/1 -> Switch/3
  Equal/1 -> Switch1/2
  Constant3/1 -> Equal/1
  Constant4/1 -> Switch1/1
  Switch2/1 -> Switch1/3
  Equal1/1 -> Switch2/2
  V_ActiveLightingMode/1 -> Equal/2, Equal1/1
  Constant2/1 -> Equal1/2
  Constant1/1 -> Switch2/1
  Constant6/1 -> Switch2/3

== system Integ_Model_Hepta/Subsystem/Slave/Function-Call Subsystem1 ==
  V_RequestedScenarioNum : Inport
  function : TriggerPort  TriggerType=function-call  VariantControl=Variant
  Constant : Constant  Value=C_IndexOfStartStepForEachScenario
  Constant1 : Constant  Value=C_NumOfStepsForEachScenario
  Constant10 : Constant  Value=C_AnimationOnLoop
  Constant11 : Constant  Value=C_MaintainAnimationPwm
  Constant12 : Constant  Value=C_MaintainAnimationTime
  Constant2 : Constant  Value=C_TStart
  Constant3 : Constant  Value=C_TRamp
  Constant4 : Constant  Value=C_EndValues
  Constant5 : Constant  Value=C_StartValues
  Constant6 : Constant  Value=C_DefaultValue
  Constant7 : Constant  Value=C_CieCurvePwmToGammaY
  Constant8 : Constant  Value=C_CieCurveGammaToPwmY
  Constant9 : Constant  Value=C_AnimationPeriod
  StdAnimationExecution : StdAnimationLibrary_R2020b/StdAnimationExecution  SystemSampleTime=-1  VariantActivationTime=update diagram  Latency=0  AutoFrameSizeCalculation=off
  Terminator1 : Terminator
  Terminator2 : Terminator
  V_AnimationPwm : Outport  VectorParamsAs1DForOutWhenUnconnected=off
  V_AnimationFinished : Outport  Port=2  VectorParamsAs1DForOutWhenUnconnected=off
  wires:
  Constant2/1 -> StdAnimationExecution/7
  Constant10/1 -> StdAnimationExecution/4
  Constant9/1 -> StdAnimationExecution/14
  Constant/1 -> StdAnimationExecution/2
  Constant6/1 -> StdAnimationExecution/11
  Constant7/1 -> StdAnimationExecution/12
  Constant4/1 -> StdAnimationExecution/9
  Constant8/1 -> StdAnimationExecution/13
  Constant3/1 -> StdAnimationExecution/8
  Constant12/1 -> StdAnimationExecution/6
  Constant11/1 -> StdAnimationExecution/5
  Constant5/1 -> StdAnimationExecution/10
  Constant1/1 -> StdAnimationExecution/3
  V_RequestedScenarioNum/1 -> StdAnimationExecution/1
  StdAnimationExecution/1 -> V_AnimationPwm/1
  StdAnimationExecution/4 -> Terminator2/1
  StdAnimationExecution/3 -> Terminator1/1
  StdAnimationExecution/2 -> V_AnimationFinished/1

== system Integ_Model_Hepta/Subsystem/Slave/Signaling ==
  C_PlOverDRL : Inport
  C_Config : Inport  Port=2
  V_PL_Rqst : Inport  Port=3
  V_CmdDrl : Inport  Port=4
  V_TI_Rqst : Inport  Port=5
  V_ActivePowerSupply : Inport  Port=6
  V_TiCycle : Inport  Port=7
  function : TriggerPort  TriggerType=function-call  VariantControl=Variant
  C_TickTIBlk : Constant  Value=C_TickTIBlk
  DrlPl : Subsystem
  Signaling1 : STD_Signaling_Lib/Signaling  SystemSampleTime=-1  VariantActivationTime=update diagram  Latency=0  AutoFrameSizeCalculation=off
  SignalsCorrected : Subsystem
  Terminator2 : Terminator
  Ti : Subsystem
  V_DrlPlFunctionTpsPwm : Outport
  V_TiFunctionTpsPwm : Outport  Port=2
  V_PL_OUT : Outport  Port=3
  V_DRL_OUT : Outport  Port=4
  wires:
  C_PlOverDRL/1 -> Signaling1/4
  C_Config/1 -> Signaling1/6
  C_TickTIBlk/1 -> Signaling1/5
  Signaling1/4 -> Terminator2/1
  DrlPl/1(V_DrlPlTpsPwm) -> V_DrlPlFunctionTpsPwm/1
  Ti/1(V_TiTpsPwm) -> V_TiFunctionTpsPwm/1
  Signaling1/3 -> Ti/1(Ti)
  V_CmdDrl/1 -> SignalsCorrected/1("V_CmdDrl ")
  V_PL_Rqst/1 -> SignalsCorrected/5(V_PL_Rqst)
  V_TI_Rqst/1 -> SignalsCorrected/2(V_CmdTi)
  V_ActivePowerSupply/1 -> SignalsCorrected/3(V_ActivePowerSupply)
  V_TiCycle/1 -> SignalsCorrected/4(V_TiCycle)
  SignalsCorrected/3(CmdTi) -> Signaling1/3
  SignalsCorrected/2(CmdDrl) -> Signaling1/2
  SignalsCorrected/1(CmdPl) -> Signaling1/1
  Signaling1/2 -> V_DRL_OUT/1, DrlPl/2(Drl)
  Signaling1/1 -> V_PL_OUT/1, DrlPl/1(Pl)

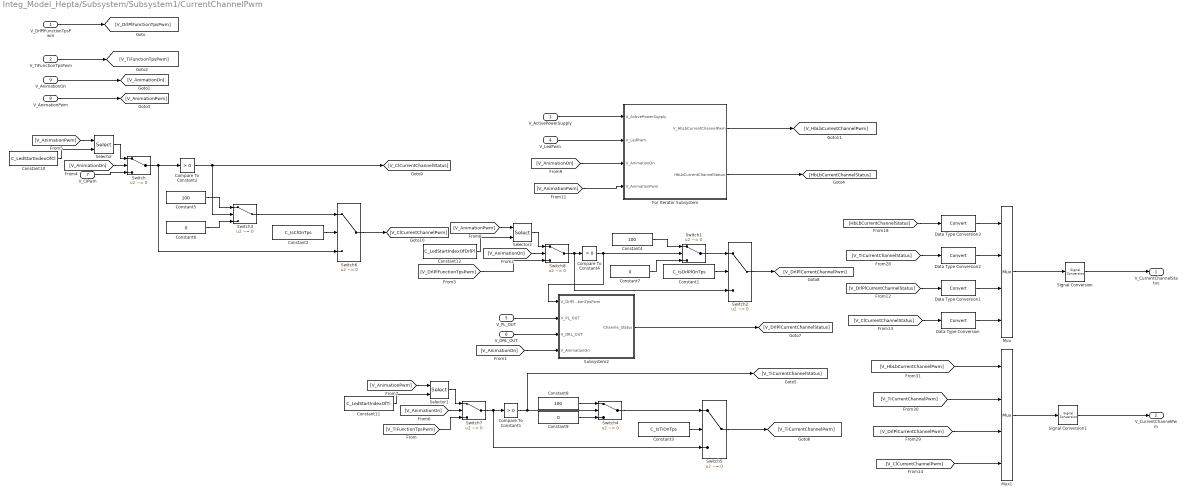
== system Integ_Model_Hepta/Subsystem/Subsystem1/CurrentChannelPwm ==
  V_DrlPlFunctionTpsPwm : Inport
  V_TiFunctionTpsPwm : Inport  Port=2
  V_ActivePowerSupply : Inport  Port=3
  V_LedPwm : Inport  Port=4
  V_PL_OUT : Inport  Port=5
  V_DRL_OUT : Inport  Port=6
  V_ClPwm : Inport  Port=7
  V_AnimationPwm : Inport  Port=8
  V_AnimationOn : Inport  Port=9
  Compare To Constant1 : simulink/Logic and Bit Operations/Compare To Constant  relop=>  const=0  OutDataTypeStr=boolean
  Compare To Constant2 : simulink/Logic and Bit Operations/Compare To Constant  relop=>  const=0  OutDataTypeStr=boolean
  Compare To Constant4 : simulink/Logic and Bit Operations/Compare To Constant  relop=>  const=0  OutDataTypeStr=boolean
  Constant1 : Constant  Value=C_IsDrlPlOnTps
  Constant10 : Constant  Value=C_LedStartIndexOfCl  OutDataTypeStr=uint8
  Constant11 : Constant  Value=C_LedStartIndexOfTi  OutDataTypeStr=uint8
  Constant12 : Constant  Value=C_LedStartIndexOfDrlPl  OutDataTypeStr=uint8
  Constant2 : Constant  Value=C_IsClOnTps
  Constant3 : Constant  Value=C_IsTiOnTps
  Constant4 : Constant  Value=100  OutDataTypeStr=Inherit: Inherit via back propagation
  Constant5 : Constant  Value=100  OutDataTypeStr=Inherit: Inherit via back propagation
  Constant6 : Constant  Value=0  OutDataTypeStr=Inherit: Inherit via back propagation
  Constant7 : Constant  Value=0  OutDataTypeStr=Inherit: Inherit via back propagation
  Constant8 : Constant  Value=100  OutDataTypeStr=Inherit: Inherit via back propagation
  Constant9 : Constant  Value=0  OutDataTypeStr=Inherit: Inherit via back propagation
  Data Type Conversion{,1..3} (4 alike) : DataTypeConversion  SaturateOnIntegerOverflow=off  RndMeth=Floor
  For Iterator Subsystem : Subsystem  TreatAsAtomicUnit=on
  Mux : Mux
  Mux1 : Mux
  Selector : Selector  IndexMode=Zero-based  IndexOptions=Index vector (port)  Indices=[1 3]  OutputSizes=1
  Selector1 : Selector  IndexMode=Zero-based  IndexOptions=Index vector (port)  Indices=[1 3]  OutputSizes=1
  Selector2 : Selector  IndexMode=Zero-based  IndexOptions=Index vector (port)  Indices=[1 3]  OutputSizes=1
  Signal Conversion : SignalConversion  OverrideOpt=off
  Signal Conversion1 : SignalConversion  OverrideOpt=off
  Subsystem2 : Subsystem
  Switch{,2,5..8} (6 alike) : Switch  Criteria=u2 ~= 0  SaturateOnIntegerOverflow=off  InputSameDT=off
  Switch1 : Switch  Criteria=u2 ~= 0  OutDataTypeStr=Inherit: Inherit via back propagation  SaturateOnIntegerOverflow=off  InputSameDT=off
  Switch3 : Switch  Criteria=u2 ~= 0  OutDataTypeStr=Inherit: Inherit via back propagation  SaturateOnIntegerOverflow=off  InputSameDT=off
  Switch4 : Switch  Criteria=u2 ~= 0  OutDataTypeStr=Inherit: Inherit via back propagation  SaturateOnIntegerOverflow=off  InputSameDT=off
  V_CurrentChannelStatus : Outport
  V_CurrentChannelPwm : Outport  Port=2
  wires:
  Constant1/1 -> Switch2/2
  Switch8/1 -> Switch2/3, Compare To Constant4/1
  Constant4/1 -> Switch1/1
  Switch1/1 -> Switch2/1
  Switch2/1 -> [V_DrlPlCurrentChannelPwm]
  Constant3/1 -> Switch5/2
  Switch4/1 -> Switch5/1
  Constant8/1 -> Switch4/1
  Constant9/1 -> Switch4/3
  Constant7/1 -> Switch1/3
  Switch5/1 -> [V_TiCurrentChannelPwm]
  V_DrlPlFunctionTpsPwm/1 -> [V_DrlPlFunctionTpsPwm]
  V_ActivePowerSupply/1 -> For Iterator Subsystem/1(V_ActivePowerSupply)
  For Iterator Subsystem/1(V_HbLbCurrentChannelPwm) -> [V_HbLbCurrentChannelPwm]
  Compare To Constant1/1 -> [V_TiCurrentChannelStatus], Switch4/2
  Subsystem2/1(Channle_Status) -> [V_DrlPlCurrentChannelStatus]
  Compare To Constant4/1 -> Switch1/2, Subsystem2/1(V_DrlPlFunctionTpsPwm)
  V_PL_OUT/1 -> Subsystem2/2(V_PL_OUT)
  [V_DrlPlFunctionTpsPwm] -> Switch8/3
  V_DRL_OUT/1 -> Subsystem2/3(V_DRL_OUT)
  For Iterator Subsystem/2(HbLbCurrentChannelStatus) -> [HbLbCurrentChannelStatus]
  V_TiFunctionTpsPwm/1 -> [V_TiFunctionTpsPwm]
  Constant6/1 -> Switch3/3
  Switch6/1 -> [V_ClCurrentChannelPwm]
  Switch3/1 -> Switch6/1
  Constant5/1 -> Switch3/1
  Constant2/1 -> Switch6/2
  Compare To Constant2/1 -> [V_ClCurrentChannelStatus], Switch3/2
  V_AnimationOn/1 -> [V_AnimationOn]
  V_AnimationPwm/1 -> [V_AnimationPwm]
  Switch/1 -> Switch6/3, Compare To Constant2/1
  [V_AnimationOn] -> Switch/2
  V_ClPwm/1 -> Switch/3
  [V_AnimationPwm] -> Selector/1
  Selector/1 -> Switch/1
  Constant10/1 -> Selector/2
  [V_AnimationPwm] -> Selector1/1
  Selector1/1 -> Switch7/1
  [V_AnimationOn] -> Switch7/2
  Constant11/1 -> Selector1/2
  [V_TiFunctionTpsPwm] -> Switch7/3
  Switch7/1 -> Switch5/3, Compare To Constant1/1
  [V_AnimationPwm] -> Selector2/1
  Selector2/1 -> Switch8/1
  [V_AnimationOn] -> Switch8/2
  Constant12/1 -> Selector2/2
  [V_AnimationOn] -> Subsystem2/4(V_AnimationOn)
  V_LedPwm/1 -> For Iterator Subsystem/2(V_LedPwm)
  [V_AnimationOn] -> For Iterator Subsystem/3(V_AnimationOn)
  [V_AnimationPwm] -> For Iterator Subsystem/4(V_AnimationPwm)
  Data Type Conversion/1 -> Mux/4
  Data Type Conversion3/1 -> Mux/1
  [V_ClCurrentChannelStatus] -> Data Type Conversion/1
  [V_DrlPlCurrentChannelStatus] -> Data Type Conversion1/1
  [V_TiCurrentChannelStatus] -> Data Type Conversion2/1
  [HbLbCurrentChannelStatus] -> Data Type Conversion3/1
  Mux1/1 -> Signal Conversion1/1
  [V_ClCurrentChannelPwm] -> Mux1/4
  [V_TiCurrentChannelPwm] -> Mux1/2
  [V_HbLbCurrentChannelPwm] -> Mux1/1
  [V_DrlPlCurrentChannelPwm] -> Mux1/3
  Mux/1 -> Signal Conversion/1
  Signal Conversion/1 -> V_CurrentChannelStatus/1
  Signal Conversion1/1 -> V_CurrentChannelPwm/1
  Data Type Conversion2/1 -> Mux/2
  Data Type Conversion1/1 -> Mux/3

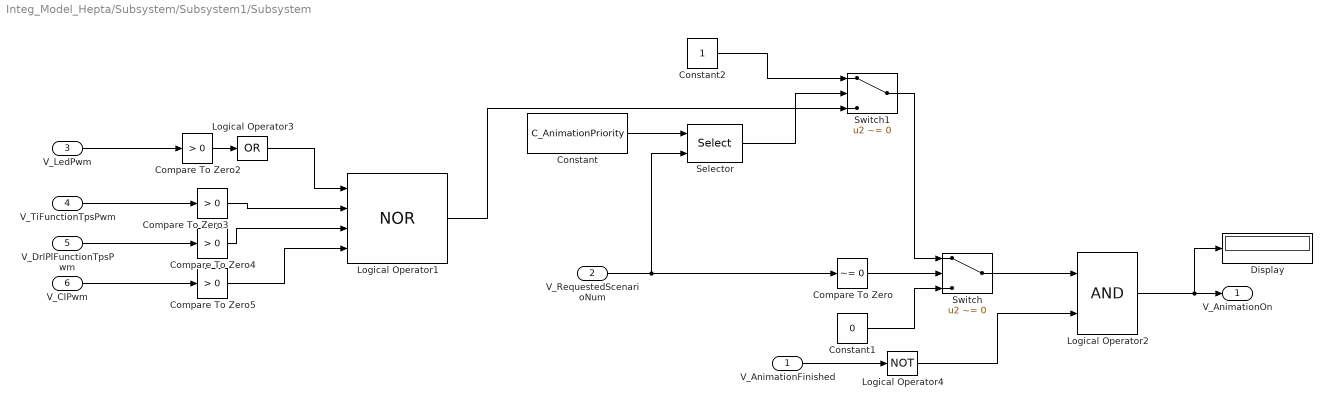
== system Integ_Model_Hepta/Subsystem/Subsystem1/Subsystem ==
  V_AnimationFinished : Inport
  V_RequestedScenarioNum : Inport  Port=2
  V_LedPwm : Inport  Port=3
  V_TiFunctionTpsPwm : Inport  Port=4
  V_DrlPlFunctionTpsPwm : Inport  Port=5
  V_ClPwm : Inport  Port=6
  Compare To Zero : simulink/Logic and Bit Operations/Compare To Zero  relop=~=  OutDataTypeStr=boolean
  Compare To Zero{2..5} (4 alike) : simulink/Logic and Bit Operations/Compare To Zero  relop=>  OutDataTypeStr=boolean
  Constant : Constant  Value=C_AnimationPriority
  Constant1 : Constant  Value=0  OutDataTypeStr=Inherit: Inherit via back propagation
  Constant2 : Constant  OutDataTypeStr=Inherit: Inherit via back propagation
  Display : Display
  Logical Operator1 : Logic  Operator=NOR  Inputs=4  AllPortsSameDT=off  OutDataTypeStr=boolean
  Logical Operator2 : Logic  AllPortsSameDT=off  OutDataTypeStr=boolean
  Logical Operator3 : Logic  Operator=OR  Inputs=1  AllPortsSameDT=off  OutDataTypeStr=boolean
  Logical Operator4 : Logic  Operator=NOT  Inputs=1  AllPortsSameDT=off  OutDataTypeStr=boolean
  Selector : Selector  IndexOptions=Index vector (port)  Indices=[1 3]  OutputSizes=1
  Switch : Switch  Criteria=u2 ~= 0  SaturateOnIntegerOverflow=off  InputSameDT=off
  Switch1 : Switch  Criteria=u2 ~= 0  SaturateOnIntegerOverflow=off  InputSameDT=off
  V_AnimationOn : Outport  VectorParamsAs1DForOutWhenUnconnected=off
  wires:
  Switch/1 -> Logical Operator2/1
  Switch1/1 -> Switch/1
  Logical Operator1/1 -> Switch1/3
  Compare To Zero/1 -> Switch/2
  V_RequestedScenarioNum/1 -> Selector/2, Compare To Zero/1
  Selector/1 -> Switch1/2
  Logical Operator4/1 -> Logical Operator2/2
  Constant1/1 -> Switch/3
  Constant2/1 -> Switch1/1
  Constant/1 -> Selector/1
  V_AnimationFinished/1 -> Logical Operator4/1
  V_DrlPlFunctionTpsPwm/1 -> Compare To Zero4/1
  V_TiFunctionTpsPwm/1 -> Compare To Zero3/1
  V_ClPwm/1 -> Compare To Zero5/1
  Logical Operator2/1 -> Display/1, V_AnimationOn/1
  V_LedPwm/1 -> Compare To Zero2/1
  Logical Operator3/1 -> Logical Operator1/1
  Compare To Zero2/1 -> Logical Operator3/1
  Compare To Zero3/1 -> Logical Operator1/2
  Compare To Zero4/1 -> Logical Operator1/3
  Compare To Zero5/1 -> Logical Operator1/4

== system Integ_Model_Hepta/Subsystem/Subsystem1/Subsystem1 ==
  HbAndLbLedPwm : Inport
  TiLedPwm : Inport  Port=2
  DrlPlLedPwm : Inport  Port=3
  ClLedPwm : Inport  Port=4
  V_AnimationOn : Inport  Port=5
  V_AnimationPwm : Inport  Port=6
  Mux : Mux
  Signal Conversion : SignalConversion  OverrideOpt=off
  Switch : Switch  Criteria=u2 > Threshold  SaturateOnIntegerOverflow=off  InputSameDT=off
  V_TpsPwm : Outport
  wires:
  TiLedPwm/1 -> Mux/2
  DrlPlLedPwm/1 -> Mux/3
  HbAndLbLedPwm/1 -> Mux/1
  ClLedPwm/1 -> Mux/4
  Mux/1 -> Switch/3
  Signal Conversion/1 -> V_TpsPwm/1
  V_AnimationPwm/1 -> Switch/1
  V_AnimationOn/1 -> Switch/2
  Switch/1 -> Signal Conversion/1

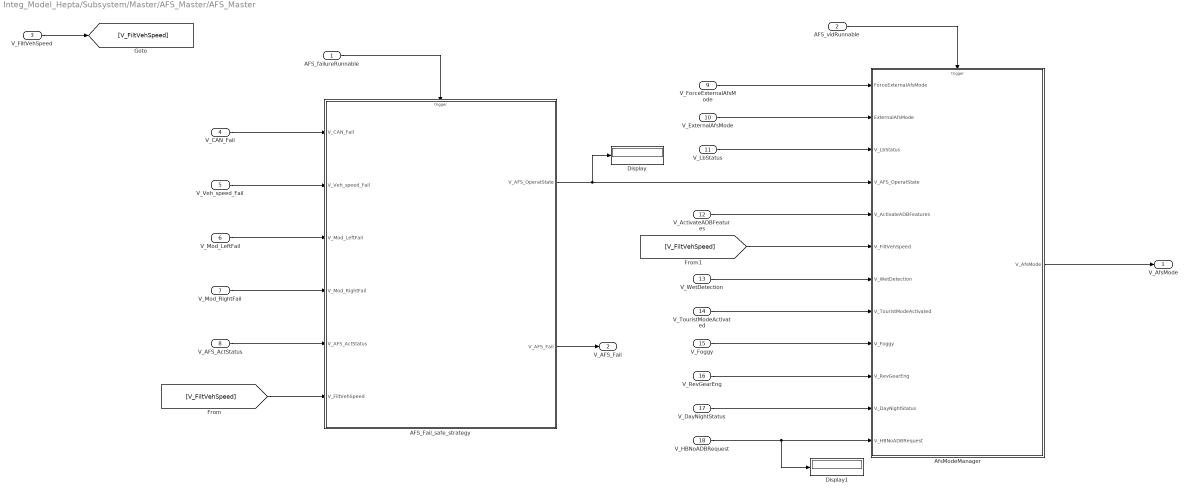
== system Integ_Model_Hepta/Subsystem/Master/AFS_Master/AFS_Master ==
  AFS_failureRunnable : Inport  OutputFunctionCall=on
  AFS_vidRunnable : Inport  Port=2  OutputFunctionCall=on
  V_FiltVehSpeed : Inport  Port=3
  V_CAN_Fail : Inport  Port=4
  V_Veh_speed_Fail : Inport  Port=5
  V_Mod_LeftFail : Inport  Port=6
  V_Mod_RightFail : Inport  Port=7
  V_AFS_ActStatus : Inport  Port=8
  V_ForceExternalAfsMode : Inport  Port=9
  V_ExternalAfsMode : Inport  Port=10
  V_LbStatus : Inport  Port=11
  V_ActivateADBFeatures : Inport  Port=12
  V_WetDetection : Inport  Port=13
  V_TouristModeActivated : Inport  Port=14
  V_Foggy : Inport  Port=15
  V_RevGearEng : Inport  Port=16
  V_DayNightStatus : Inport  Port=17
  V_HBNoADBRequest : Inport  Port=18
  AFS_Fail_safe_strategy : Subsystem  Description=AFS_Fail_safe_strategy
  AfsModeManager : Subsystem  Description=AfsModeManager
  Display : Display
  Display1 : Display
  V_AfsMode : Outport  PortDimensions=1
  V_AFS_Fail : Outport  Port=2  VectorParamsAs1DForOutWhenUnconnected=off
  wires:
  V_TouristModeActivated/1 -> AfsModeManager/8(V_TouristModeActivated)
  V_ActivateADBFeatures/1 -> AfsModeManager/5(V_ActivateADBFeatures)
  V_ExternalAfsMode/1 -> AfsModeManager/2(ExternalAfsMode)
  V_RevGearEng/1 -> AfsModeManager/10(V_RevGearEng)
  AfsModeManager/1(V_AfsMode) -> V_AfsMode/1
  V_WetDetection/1 -> AfsModeManager/7(V_WetDetection)
  V_LbStatus/1 -> AfsModeManager/3(V_LbStatus)
  V_ForceExternalAfsMode/1 -> AfsModeManager/1(ForceExternalAfsMode)
  V_Foggy/1 -> AfsModeManager/9(V_Foggy)
  AFS_vidRunnable/1 -> AfsModeManager/Trigger
  V_CAN_Fail/1 -> AFS_Fail_safe_strategy/1(V_CAN_Fail)
  V_Veh_speed_Fail/1 -> AFS_Fail_safe_strategy/2(V_Veh_speed_Fail)
  AFS_failureRunnable/1 -> AFS_Fail_safe_strategy/Trigger
  V_AFS_ActStatus/1 -> AFS_Fail_safe_strategy/5(V_AFS_ActStatus)
  V_FiltVehSpeed/1 -> [V_FiltVehSpeed]
  [V_FiltVehSpeed] -> AFS_Fail_safe_strategy/6(V_FiltVehSpeed)
  [V_FiltVehSpeed] -> AfsModeManager/6(V_FiltVehSpeed)
  AFS_Fail_safe_strategy/2(V_AFS_Fail) -> V_AFS_Fail/1
  V_Mod_LeftFail/1 -> AFS_Fail_safe_strategy/3(V_Mod_LeftFail)
  V_Mod_RightFail/1 -> AFS_Fail_safe_strategy/4(V_Mod_RightFail)
  AFS_Fail_safe_strategy/1(V_AFS_OperatState) -> Display/1, AfsModeManager/4(V_AFS_OperatState)
  V_DayNightStatus/1 -> AfsModeManager/11(V_DayNightStatus)
  V_HBNoADBRequest/1 -> Display1/1, AfsModeManager/12(V_HBNoADBRequest)

== system Integ_Model_Hepta/Subsystem/Master/Cl_Master/CL_MasterFunction ==
  V_TiLeft : Inport
  V_TiRight : Inport  Port=2
  V_FiltVehSpeed : Inport  Port=3
  V_CurveRadius : Inport  Port=4
  V_FiltStWhAngleScaled : Inport  Port=5
  function : TriggerPort  TriggerType=function-call  VariantControl=Variant
  Cl_Master_func_Call : Subsystem
  V_ClRight : Outport
  V_ClLeft : Outport  Port=2
  wires:
  V_FiltVehSpeed/1 -> Cl_Master_func_Call/3(V_FiltVehSpeed)
  V_CurveRadius/1 -> Cl_Master_func_Call/4(V_CurveRadius)
  V_TiLeft/1 -> Cl_Master_func_Call/1(V_TiLeft)
  V_TiRight/1 -> Cl_Master_func_Call/2(V_TiRight)
  V_FiltStWhAngleScaled/1 -> Cl_Master_func_Call/5(V_FiltStWhAngleScaled)
  Cl_Master_func_Call/2(V_ClLeft) -> V_ClLeft/1
  Cl_Master_func_Call/1(V_ClRight) -> V_ClRight/1
